simulink model "test_case_generator"  (R2015b)
settings: Solver=ode4  StartTime=0.0  StopTime=10.0  FixedStep=0.1  RelTol=1e-3
undefined symbols (not defined in the file or in its folder): sigbuilder_block
settings Model: Creator=nctzv8  LastModifiedBy=nctzv8

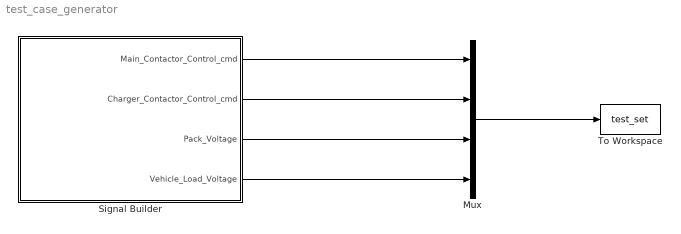
== system test_case_generator ==
  Mux : Mux
  Signal Builder : Subsystem  Tag=STV Subsys  LoadFcn=sigbuilder_block('load');  StartFcn=sigbuilder_block('start');  StopFcn=sigbuilder_block('stop');  ClipboardFcn=sigbuilder_block('clipboard');  mask(Sigbuilder block){}
      mask help: Simulink:masks:SigbuilderBlock_MD
      mask init:
      | if ~strcmp(get_param(bdroot(gcbh),'SimulationStatus'),'stopped') tuvar = sigbuilder_block('maskInit'); end
      settings: CopyFcn=sigbuilder_block('copy');  DeleteFcn=sigbuilder_block('delete');  ModelCloseFcn=sigbuilder_block('modelClose');  PreSaveFcn=sigbuilder_block('preSave');  PauseFcn=sigbuilder_block('pause');  ContinueFcn=sigbuilder_block('continue');  NameChangeFcn=sigbuilder_block('namechange');  OpenFcn=sigbuilder_block('open',[5.4 30 1141.2 522.6 ]);  CloseFcn=sigbuilder_block('close');
      mask Display: plot(0, 0, 100, 100,[2, 2, 32, 32, 2], [68, 8, 8, 68, 68],[32, 2], [38, 38], [32, 19, 2],[53, 60, 44], [32, 17, 17, 2],[16, 16, 31, 31]);txt = getActiveGroup(gcbh);text(2, 100, txt,'verticalAlignment', 'top');
  To Workspace : ToWorkspace  VariableName=test_set  SaveFormat=Timeseries  SampleTime=-1
  wires:
  Mux/1 -> To Workspace/1
  Signal Builder/1(Main_Contactor_Control_cmd) -> Mux/1
  Signal Builder/2(Charger_Contactor_Control_cmd) -> Mux/2
  Signal Builder/3(Pack_Voltage) -> Mux/3
  Signal Builder/4(Vehicle_Load_Voltage) -> Mux/4

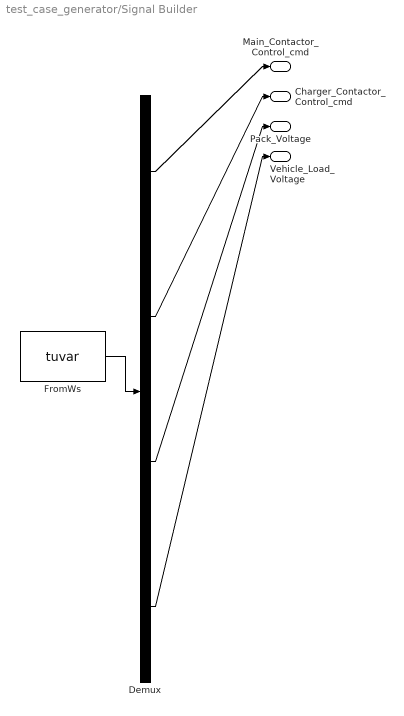
== system test_case_generator/Signal Builder ==
  Demux : Demux  Tag=STV Demux
  FromWs : FromWorkspace  Tag=STV FromWs  VariableName=tuvar  SampleTime=0
      SigBuilderData=|
      | common.afterFinalStr = 'Extrapolate'
      | common.sampleTime = 0
      | dataSet(1).timeRange = [0 10]
      | dataSet(1).name = 'TS1'
      | dataSet(2).timeRange = [0 10]
      | dataSet(2).name = 'TS2'
      | dataSet(3).timeRange = [0 10]
      | dataSet(3).name = 'TS3'
      | dataSet(4).timeRange = [0 10]
      | dataSet(4).name = 'TS4'
      | dataSet(5).timeRange = [0 10]
      | dataSet(5).name = 'TS5'
      | sbobj.Groups(1).Name = 'TS1'
      | sbobj.Groups(1).Signals(1).Name = 'Main_Contactor_Control_cmd'
      | sbobj.Groups(1).Signals(1).XData = [0 1 1 6 10]
      | sbobj.Groups(1).Signals(1).YData = [0 0 1 1 1]
      | sbobj.Groups(1).Signals(2).Name = 'Charger_Contactor_Control_cmd'
      | sbobj.Groups(1).Signals(2).XData = [0 4 6.51 7.51 10]
      | sbobj.Groups(1).Signals(2).YData = [0 0 0 0 0]
      | sbobj.Groups(1).Signals(3).Name = 'Pack_Voltage'
      | sbobj.Groups(1).Signals(3).XData = [0 7 10]
      | sbobj.Groups(1).Signals(3).YData = [140 140 140]
      | sbobj.Groups(1).Signals(4).Name = 'Vehicle_Load_Voltage'
      | sbobj.Groups(1).Signals(4).XData = [0 1 1.2 7 10]
      | sbobj.Groups(1).Signals(4).YData = [0 0 140 140 140]
      | sbobj.Groups(2).Name = 'TS2'
      | sbobj.Groups(2).Signals(1).Name = 'Main_Contactor_Control_cmd'
      | sbobj.Groups(2).Signals(1).XData = [0 1 6 10]
      | sbobj.Groups(2).Signals(1).YData = [0 0 0 0]
      | sbobj.Groups(2).Signals(2).Name = 'Charger_Contactor_Control_cmd'
      | sbobj.Groups(2).Signals(2).XData = [0 1 1 7.51 10]
      | sbobj.Groups(2).Signals(2).YData = [0 0 1 1 1]
      | sbobj.Groups(2).Signals(3).Name = 'Pack_Voltage'
      | sbobj.Groups(2).Signals(3).XData = [0 7 10]
      | sbobj.Groups(2).Signals(3).YData = [140 140 140]
      | sbobj.Groups(2).Signals(4).Name = 'Vehicle_Load_Voltage'
      | sbobj.Groups(2).Signals(4).XData = [0 1 1.2 7 10]
      | sbobj.Groups(2).Signals(4).YData = [0 0 140 140 140]
      | sbobj.Groups(3).Name = 'TS3'
      | sbobj.Groups(3).Signals(1).Name = 'Main_Contactor_Control_cmd'
      | sbobj.Groups(3).Signals(1).XData = [0 1 1 6 6 10]
      | sbobj.Groups(3).Signals(1).YData = [0 0 1 1 0 0]
      | sbobj.Groups(3).Signals(2).Name = 'Charger_Contactor_Control_cmd'
      | sbobj.Groups(3).Signals(2).XData = [0 4 6.51 7.51 10]
      | sbobj.Groups(3).Signals(2).YData = [0 0 0 0 0]
      | sbobj.Groups(3).Signals(3).Name = 'Pack_Voltage'
      | sbobj.Groups(3).Signals(3).XData = [0 7 10]
      | sbobj.Groups(3).Signals(3).YData = [140 140 140]
      | sbobj.Groups(3).Signals(4).Name = 'Vehicle_Load_Voltage'
      | sbobj.Groups(3).Signals(4).XData = [0 1 1.2 7 10]
      | sbobj.Groups(3).Signals(4).YData = [0 0 140 140 140]
      | sbobj.Groups(4).Name = 'TS4'
      | sbobj.Groups(4).Signals(1).Name = 'Main_Contactor_Control_cmd'
      | sbobj.Groups(4).Signals(1).XData = [0 1 6 10]
      | sbobj.Groups(4).Signals(1).YData = [0 0 0 0]
      | sbobj.Groups(4).Signals(2).Name = 'Charger_Contactor_Control_cmd'
      | sbobj.Groups(4).Signals(2).XData = [0 1 1 6 6 10]
      | sbobj.Groups(4).Signals(2).YData = [0 0 1 1 0 0]
      | sbobj.Groups(4).Signals(3).Name = 'Pack_Voltage'
      | sbobj.Groups(4).Signals(3).XData = [0 7 10]
      | sbobj.Groups(4).Signals(3).YData = [140 140 140]
      | sbobj.Groups(4).Signals(4).Name = 'Vehicle_Load_Voltage'
      | sbobj.Groups(4).Signals(4).XData = [0 1 1.2 7 10]
      | sbobj.Groups(4).Signals(4).YData = [0 0 140 140 140]
      | sbobj.Groups(5).Name = 'TS5'
      | sbobj.Groups(5).Signals(1).Name = 'Main_Contactor_Control_cmd'
      | sbobj.Groups(5).Signals(1).XData = [0 1 1 6 10]
      | sbobj.Groups(5).Signals(1).YData = [0 0 1 1 1]
      | sbobj.Groups(5).Signals(2).Name = 'Charger_Contactor_Control_cmd'
      | sbobj.Groups(5).Signals(2).XData = [0 4 6.51 7.51 10]
      | sbobj.Groups(5).Signals(2).YData = [0 0 0 0 0]
      | sbobj.Groups(5).Signals(3).Name = 'Pack_Voltage'
      | sbobj.Groups(5).Signals(3).XData = [0 7 10]
      | sbobj.Groups(5).Signals(3).YData = [140 140 140]
      | sbobj.Groups(5).Signals(4).Name = 'Vehicle_Load_Voltage'
      | sbobj.Groups(5).Signals(4).XData = [0 1 1.2 7 10]
      | sbobj.Groups(5).Signals(4).YData = [0 0 0 0 0]
  Main_Contactor_Control_cmd : Outport  Tag=STV Outport
  Charger_Contactor_Control_cmd : Outport  Tag=STV Outport  Port=2
  Pack_Voltage : Outport  Tag=STV Outport  Port=3
  Vehicle_Load_Voltage : Outport  Tag=STV Outport  Port=4
  wires:
  FromWs/1 -> Demux/1
  Demux/1 -> Main_Contactor_Control_cmd/1
  Demux/2 -> Charger_Contactor_Control_cmd/1
  Demux/3 -> Pack_Voltage/1
  Demux/4 -> Vehicle_Load_Voltage/1
